simulink model "hw2_ex5_spring"  (R2024b)
settings: Solver=VariableStepAuto  StartTime=0.0  StopTime=10.0  FixedStep=sample  RelTol=1e-3  EnableMultiTasking=on
values from neighbouring files (symbols this model uses):
  noise = 0    [ex5_1.m]    (also in ex5_2.m = 0.001)
  step_mag = 2    [ex5_1.m]    (also in ex5_2.m = step_mags(i))
  Ts = t(2)-t(1)    [ex3.m]    (also in ex4.m; ex5_1.m = 0.1; ex5_2.m = 0.1)
settings Model: Creator=hespanha  LastModifiedBy=blixo
settings SolverCC: AlgebraicLoopSolver=TrustRegion
settings DataIOCC: LimitDataPoints=on  SaveFormat=Array  SignalLoggingSaveFormat=ModelDataLogs  ReturnWorkspaceOutputs=off  SignalLoggingName=sigsOut
settings DebuggingCC: SaveWithParameterizedLinksMsg=none  UnderspecifiedInitializationDetection=Classic  MergeDetectMultiDrivingBlocksExec=none  SignalResolutionControl=TryResolveAllWithWarning  MultiTaskDSMMsg=warning  MultiTaskCondExecSysMsg=none  UnconnectedInputMsg=warning  UnconnectedOutputMsg=warning  UnconnectedLineMsg=warning  ArithmeticOperatorsInVariantConditions=warning
settings HardwareCC: ProdBitPerPointer=32  ProdBitPerSizeT=32  ProdBitPerPtrDiffT=32  ProdLargestAtomicFloat=None  ProdIntDivRoundTo=Undefined  ProdEndianess=Unspecified  ProdWordSize=32  ProdHWDeviceType=32-bit Generic  TargetUnknown=on
settings ModelReferenceCC: EnableRefExpFcnMdlSchedulingChecks=on  PropagateSignalLabelsOutOfModel=off
settings SFSimCC: CustomCodeUndefinedFunction=UseInterfaceOnly
settings RTWCC: GPUComputeCapability=3.5
settings GRTTargetCC: CombineOutputUpdateFcns=off  GRTInterface=on
settings ConfigComp: CovMetricSettings=dw  CovSaveCumulativeToWorkspaceVar=on  CovSaveSingleToWorkspaceVar=on

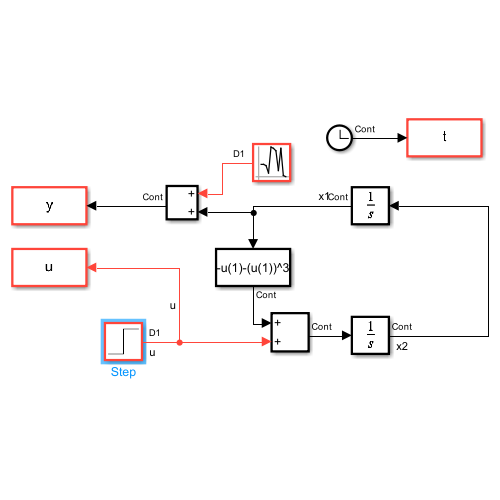
[thumbnail: Simulink's stored preview of the top-level diagram]
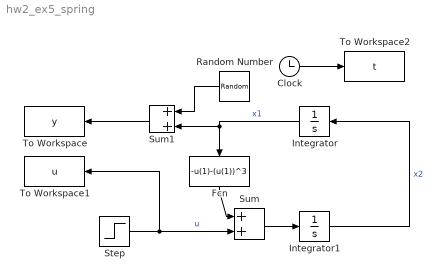
== system hw2_ex5_spring ==
  Clock : Clock
  Fcn : Fcn  Expr=-u(1)-(u(1))^3
  Integrator : Integrator
  Integrator1 : Integrator
  Random Number : RandomNumber  Variance=noise  SampleTime=Ts
  Step : Step  After=step_mag  SampleTime=Ts
  Sum : Sum  SaturateOnIntegerOverflow=on
  Sum1 : Sum  SaturateOnIntegerOverflow=on
  To Workspace : ToWorkspace  VariableName=y  SampleTime=Ts
  To Workspace1 : ToWorkspace  VariableName=u  SampleTime=Ts
  To Workspace2 : ToWorkspace  VariableName=t  SampleTime=Ts
  wires:
  Sum1/1 -> To Workspace/1
  Random Number/1 -> Sum1/1
  Step/1 -> Sum/2, To Workspace1/1  "u"
  Fcn/1 -> Sum/1
  Sum/1 -> Integrator1/1
  Integrator/1 -> Fcn/1, Sum1/2  "x1"
  Integrator1/1 -> Integrator/1  "x2"
  Clock/1 -> To Workspace2/1
